simulink model "problem3"  (R2020a)
settings: Solver=ode45  StartTime=0.0  StopTime=10  RelTol=1e-3
undefined symbols (not defined in the file): Ki, Kp
settings Model: DataDictionary=pidcontrol.sldd  Creator=Jake  LastModifiedBy=Jake

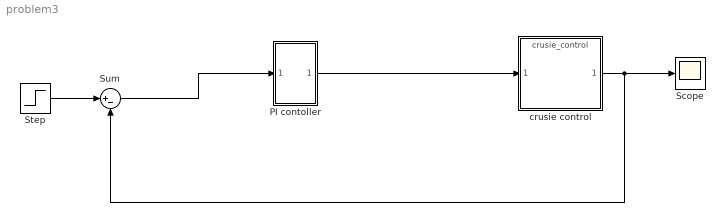
== system problem3 ==
  PI contoller : Subsystem
  Scope : Scope
  Step : Step  Time=0  After=10  SampleTime=0
  Sum : Sum  Inputs=|+-
  crusie control : ModelReference  ModelNameDialog=crusie_control  ModelReferenceVersion=1.3
  wires:
  Step/1 -> Sum/1
  crusie control/1 -> Scope/1, Sum/2
  Sum/1 -> PI contoller/1(In1)
  PI contoller/1(Out1) -> crusie control/1

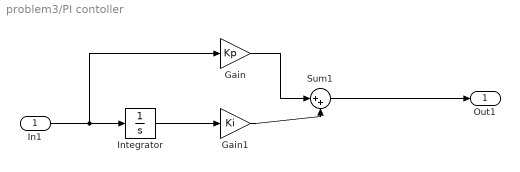
== system problem3/PI contoller ==
  In1 : Inport
  Gain : Gain  Gain=Kp
  Gain1 : Gain  Gain=Ki
  Integrator : Integrator
  Sum1 : Sum  Inputs=|++
  Out1 : Outport
  wires:
  Gain1/1 -> Sum1/2
  Sum1/1 -> Out1/1
  In1/1 -> Gain/1, Integrator/1
  Gain/1 -> Sum1/1
  Integrator/1 -> Gain1/1
